simulink model "test11"  (R2021a)
settings: Solver=VariableStepAuto  StartTime=0.0  StopTime=8  RelTol=1e-3
model workspace (MAT data in the model file):
  SDO_OutputTimes = [0 0.00347222222222 0.00694444444444 0.0104166666667 0.0138888888889 0.0173611111111 0.0208333333333 0.0243055555556 0.0277777777778 0.03125 0.0347222222222 0.0381944444444 ... (4607 elements, 4607x1)]
  params = climate_p
  params.A_f = 3100.00212382
  params.A_c = 3299.99831764
  params.minWindows = 0.499999921997
  params.alpha_i = 0.106667779901
  params.cd_c = 8999.32112543
  params.T_ss = 280.000272426
libraries: HORTISIM x3
(part 1 of 2)
settings Model: SimulationMode=accelerator  OrderedModelArguments=off  Creator=djoroya  LastModifiedBy=djoroya
settings DebuggingCC: UnconnectedInputMsg=none  UnconnectedOutputMsg=none  UnconnectedLineMsg=none

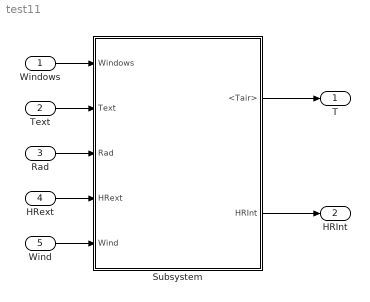
== system test11 ==
  Windows : Inport
  Text : Inport  Port=2
  Rad : Inport  Port=3
  HRext : Inport  Port=4
  Wind : Inport  Port=5
  Subsystem : Subsystem
  T : Outport
  HRInt : Outport  Port=2
  wires:
  Subsystem/1(<Tair>) -> T/1
  Windows/1 -> Subsystem/1(Windows)
  Text/1 -> Subsystem/2(Text)
  Rad/1 -> Subsystem/3(Rad)
  HRext/1 -> Subsystem/4(HRext)
  Wind/1 -> Subsystem/5(Wind)
  Subsystem/2(HRInt) -> HRInt/1
